simulink model "example_0413"  (R2022b)
settings: Solver=FixedStepAuto  StartTime=0.0  StopTime=1000.0  FixedStep=0.2  RelTol=1e-3
settings Model: Creator=33093  LastModifiedBy=33093

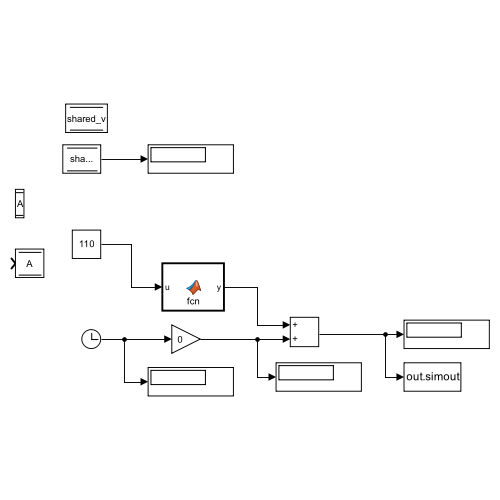
[thumbnail: Simulink's stored preview of the top-level diagram]
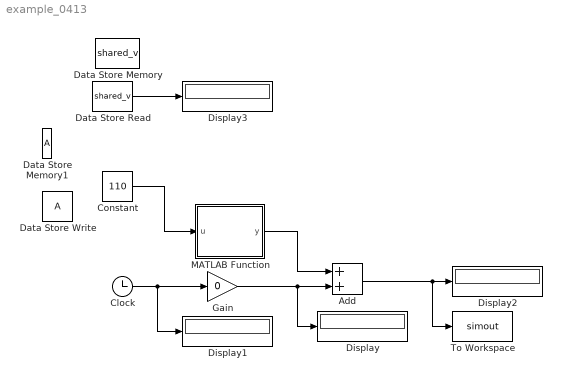
== system example_0413 ==
  Add : Sum
  Clock : Clock
  Constant : Constant  Value=110
  Data Store Memory : DataStoreMemory  DataStoreName=shared_v  WriteAfterWriteMsg=warning  InitialValue=1  ShowAdditionalParam=off  OutDataTypeStr=double
  Data Store Memory1 : DataStoreMemory  WriteAfterWriteMsg=warning  ShowAdditionalParam=off
  Data Store Read : DataStoreRead  DataStoreName=shared_v  DataStoreElements=shared_v  IndexOptions=Index vector (dialog)  Indices=1  OutputSizes=1
  Data Store Write : DataStoreWrite  IndexOptions=Index vector (dialog)  Indices=1  OutputSizes=1
  Display{,1..3} (4 alike) : Display
  Gain : Gain  Gain=0
  MATLAB Function : MATLAB Function  TreatAsAtomicUnit=on
  To Workspace : ToWorkspace  VariableName=simout  SampleTime=-1
  wires:
  Add/1 -> Display2/1, To Workspace/1
  Constant/1 -> MATLAB Function/1(u)
  Data Store Read/1 -> Display3/1
  Clock/1 -> Gain/1, Display1/1
  MATLAB Function/1(y) -> Add/1
  Gain/1 -> Add/2, Display/1

== matlab function example_0413/MATLAB Function ==
  data: u input; y output; shared_v data_store_memory; x parameter
function y = fcn(u, x)
global shared_v;
y = shared_v*x;
end
